simulink model "AdaptiveControlsProjectPart1_Sethi"  (R2019b)
settings: Solver=ode45  StartTime=0.0  StopTime=40  RelTol=1e-6
undefined symbols (not defined in the file): Ar, ar, Astar, astar, B, Br, br, Bstar, bstar, cur0, eps_th, Gam_r, gam_r, Gam_x, gam_x, J, K, L, P, P2, Q, R, th_max, thr0, thx0, Tr_star, tr_star, Tx_star, tx_star, V0, X0, x0, Xr0, xr0
settings Model: Creator=aleon  LastModifiedBy=Japnit Sethi
settings SFSimCC: CustomCodeUndefinedFunction=UseInterfaceOnly

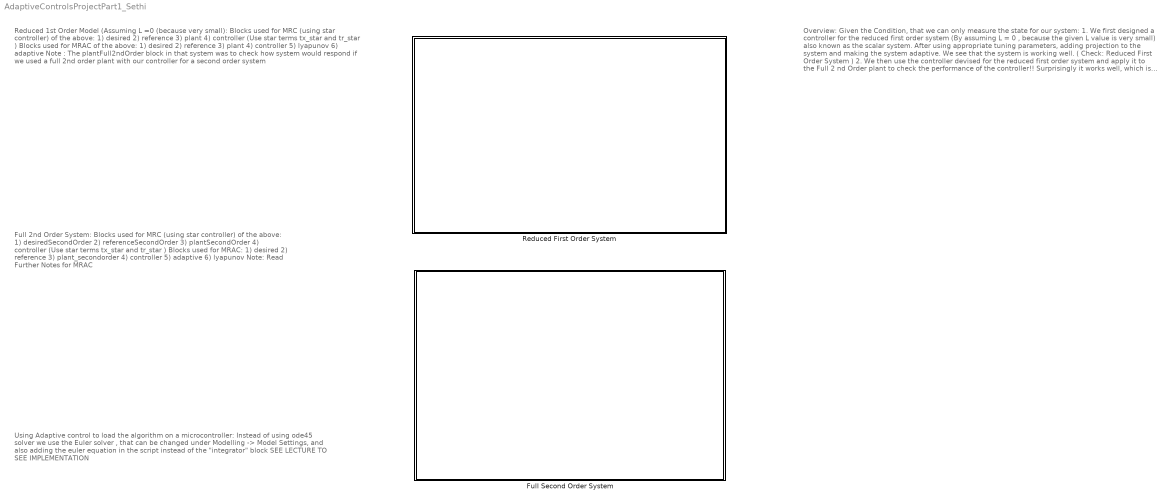
== system AdaptiveControlsProjectPart1_Sethi ==
  note: Reduced 1st Order Model (Assuming L =0 (because very small):
      |
      | Blocks used for MRC (using star controller) of the above:
      | 1) desired
      | 2) reference
      | 3) plant
      | 4) controller (Use star terms tx_star and tr_star )
      |
      | Blocks used for MRAC of the above:
      | 1) desired
      | 2) reference
      | 3) plant
      | 4) controller
      | 5) lyapunov
      | 6) adaptive
      |
      | Note : The plantFull2ndOrder block in that system was to check how system would respond if we used a full 2nd order plant with our controller for a second order system
  note: Using Adaptive control to load the algorithm on a microcontroller:
      |
      | Instead of using ode45 solver we use the Euler solver , that can be changed under Modelling -> Model Settings,
      | and also adding the euler equation in the script instead of the "integrator" block
      |
      | SEE LECTURE TO SEE IMPLEMENTATION
  note: Full 2nd Order System:
      |
      | Blocks used for MRC (using star controller) of the above:
      | 1) desiredSecondOrder
      | 2) referenceSecondOrder
      | 3) plantSecondOrder
      | 4) controller (Use star terms tx_star and tr_star )
      |
      | Blocks used for MRAC:
      | 1) desired
      | 2) reference
      | 3) plant_secondorder
      | 4) controller
      | 5) adaptive
      | 6) lyapunov
      | Note: Read Further Notes for MRAC
  note: Overview:
      | Given the Condition, that we can only measure the state for our system:
      | 1. We first designed a controller for the reduced first order system (By assuming L = 0 , because the given L value is very small) also known as the scalar system. After using appropriate tuning parameters, adding projection to the system and making the system adaptive. We see that the system is working well. ( Check: Reduced First Order System )
      | 2. We then use the controller devised for the reduced first order system and apply it to the Full 2 nd Order plant to check the performance of the controller!! Surprisingly it works well, which is because the approximation of L was legible.
      | 3. We designed a Full state feedback controller for the Full second order system, by deriving the equations in canonical form and also change our states from and to and which is important in order to derive and satisfy our compatibility equations. In this scenario, we were able to measure both and . ( Check: Full Second Order System )
      | 4. Finally, we designed a Full Output Feedback controller , because in really, we cannot measure , the only measurement available to us is .
      | Note: ( Option 2: But not recommended ) For the Full output feedback controller above, we could measure and then calculate the by computing a numerical derivative of measured and adding a filter transfer function to get rid of the noise. But this is not preferred because excessive time that we can lose tuning our parameters to get rid of high oscillations and noise.
  Full Second Order System : Subsystem
  Reduced First Order System : Subsystem

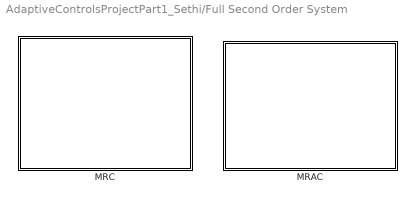
== system AdaptiveControlsProjectPart1_Sethi/Full Second Order System ==
  MRAC : Subsystem
  MRC : Subsystem

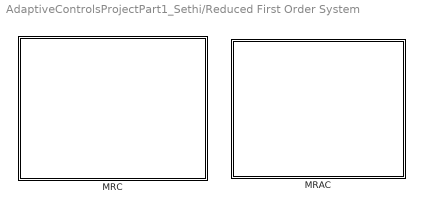
== system AdaptiveControlsProjectPart1_Sethi/Reduced First Order System ==
  MRAC : Subsystem
  MRC : Subsystem

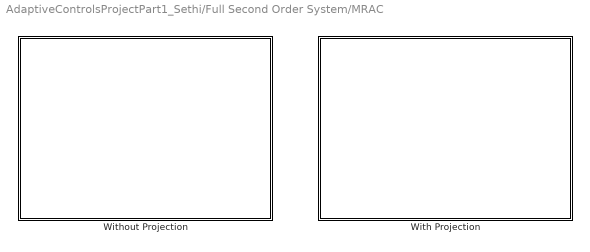
== system AdaptiveControlsProjectPart1_Sethi/Full Second Order System/MRAC ==
  With Projection : Subsystem
  Without Projection : Subsystem

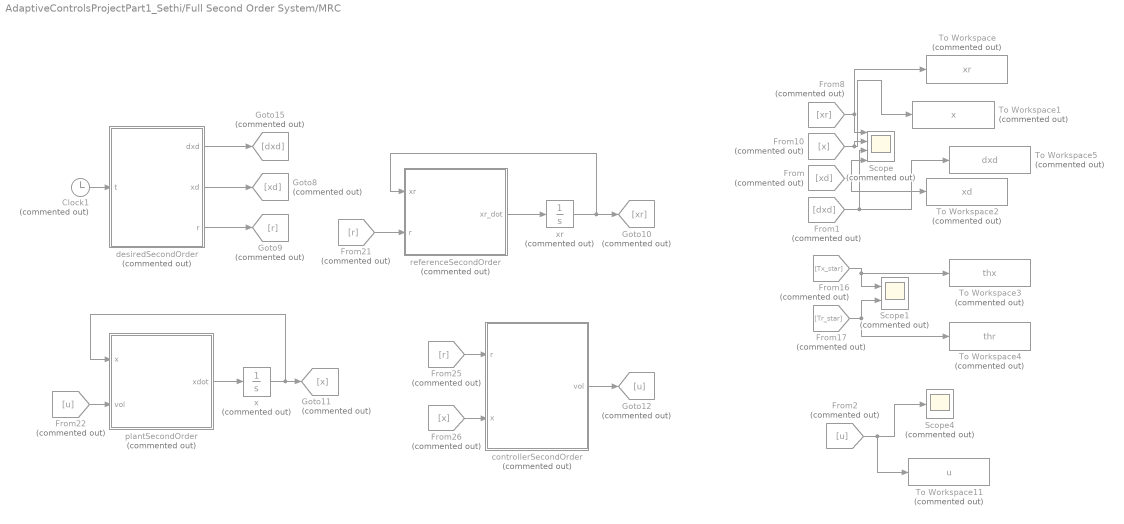
== system AdaptiveControlsProjectPart1_Sethi/Full Second Order System/MRC ==
  Clock1 : Clock  Commented=on
  From : From  Commented=on  GotoTag=xd
  From1 : From  Commented=on  GotoTag=dxd
  From10 : From  Commented=on  GotoTag=x
  From16 : From  Commented=on  GotoTag=Tx_star
  From17 : From  Commented=on  GotoTag=Tr_star
  From2 : From  Commented=on  GotoTag=u
  From21 : From  Commented=on  GotoTag=r
  From22 : From  Commented=on  GotoTag=u
  From25 : From  Commented=on  GotoTag=r
  From26 : From  Commented=on  GotoTag=x
  From8 : From  Commented=on  GotoTag=xr
  Goto10 : Goto  Commented=on  GotoTag=xr
  Goto11 : Goto  Commented=on  GotoTag=x
  Goto12 : Goto  Commented=on  GotoTag=u
  Goto15 : Goto  Commented=on  GotoTag=dxd
  Goto8 : Goto  Commented=on  GotoTag=xd
  Goto9 : Goto  Commented=on  GotoTag=r
  Scope : Scope  Commented=on  NumInputPorts=4
  Scope1 : Scope  Commented=on  NumInputPorts=2
  Scope4 : Scope  Commented=on
  To Workspace : ToWorkspace  Commented=on  VariableName=xr  SampleTime=-1
  To Workspace1 : ToWorkspace  Commented=on  VariableName=x  SampleTime=-1
  To Workspace11 : ToWorkspace  Commented=on  VariableName=u  SampleTime=-1
  To Workspace2 : ToWorkspace  Commented=on  VariableName=xd  SampleTime=-1
  To Workspace3 : ToWorkspace  Commented=on  VariableName=thx  SampleTime=-1
  To Workspace4 : ToWorkspace  Commented=on  VariableName=thr  SampleTime=-1
  To Workspace5 : ToWorkspace  Commented=on  VariableName=dxd  SampleTime=-1
  controllerSecondOrder : MATLAB Function  Commented=on  TreatAsAtomicUnit=on
  desiredSecondOrder : MATLAB Function  Commented=on  TreatAsAtomicUnit=on
  plantSecondOrder : MATLAB Function  Commented=on  TreatAsAtomicUnit=on
  referenceSecondOrder : MATLAB Function  Commented=on  TreatAsAtomicUnit=on
  x : Integrator  Commented=on  InitialCondition=X0
  xr : Integrator  Commented=on  InitialCondition=Xr0
  wires:
  desiredSecondOrder/3(r) -> Goto9/1
  From/1 -> To Workspace2/1, Scope/4
  From1/1 -> To Workspace5/1, Scope/3
  From10/1 -> To Workspace1/1, Scope/2
  x/1 -> plantSecondOrder/1(x), Goto11/1
  controllerSecondOrder/1(vol) -> Goto12/1
  From17/1 -> Scope1/2, To Workspace4/1
  From22/1 -> plantSecondOrder/2(vol)
  desiredSecondOrder/1(dxd) -> Goto15/1
  From26/1 -> controllerSecondOrder/2(x)
  Clock1/1 -> desiredSecondOrder/1(t)
  referenceSecondOrder/1(xr_dot) -> xr/1
  xr/1 -> Goto10/1, referenceSecondOrder/1(xr)
  From8/1 -> Scope/1, To Workspace/1
  From25/1 -> controllerSecondOrder/1(r)
  plantSecondOrder/1(xdot) -> x/1
  desiredSecondOrder/2(xd) -> Goto8/1
  From21/1 -> referenceSecondOrder/2(r)
  From16/1 -> To Workspace3/1, Scope1/1
  From2/1 -> To Workspace11/1, Scope4/1

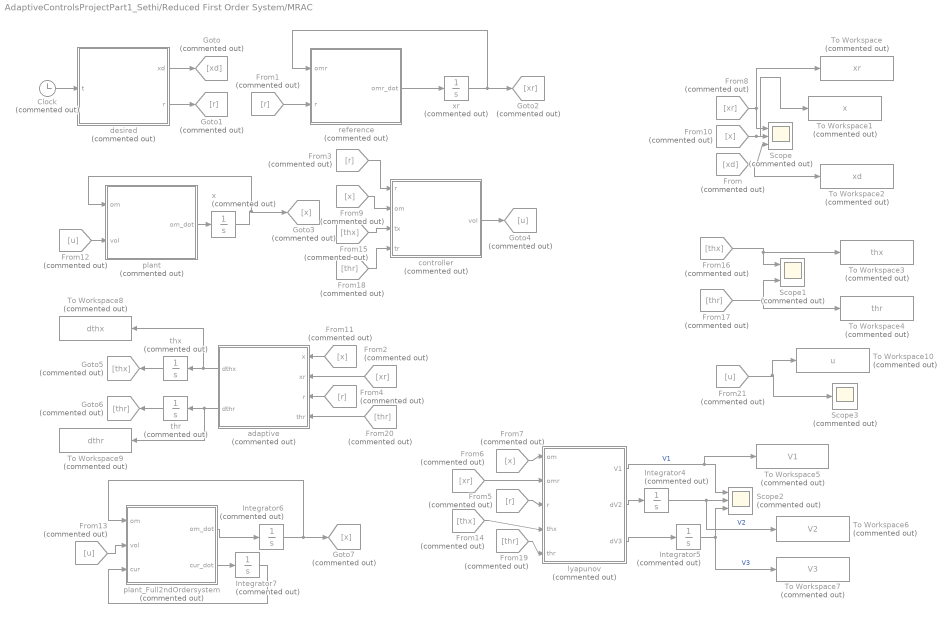
== system AdaptiveControlsProjectPart1_Sethi/Reduced First Order System/MRAC ==
  Clock : Clock  Commented=on
  From : From  Commented=on  GotoTag=xd
  From{1,3..5} (4 alike) : From  Commented=on  GotoTag=r
  From{7,9..11} (4 alike) : From  Commented=on  GotoTag=x
  From12 : From  Commented=on  GotoTag=u
  From13 : From  Commented=on  GotoTag=u
  From14 : From  Commented=on  GotoTag=thx
  From15 : From  Commented=on  GotoTag=thx
  From16 : From  Commented=on  GotoTag=thx
  From{17..20} (4 alike) : From  Commented=on  GotoTag=thr
  From2 : From  Commented=on  GotoTag=xr
  From21 : From  Commented=on  GotoTag=u
  From6 : From  Commented=on  GotoTag=xr
  From8 : From  Commented=on  GotoTag=xr
  Goto : Goto  Commented=on  GotoTag=xd
  Goto1 : Goto  Commented=on  GotoTag=r
  Goto2 : Goto  Commented=on  GotoTag=xr
  Goto3 : Goto  Commented=on  GotoTag=x
  Goto4 : Goto  Commented=on  GotoTag=u
  Goto5 : Goto  Commented=on  GotoTag=thx
  Goto6 : Goto  Commented=on  GotoTag=thr
  Goto7 : Goto  Commented=on  GotoTag=x
  Integrator4 : Integrator  Commented=on  InitialCondition=V0
  Integrator5 : Integrator  Commented=on  InitialCondition=V0
  Integrator6 : Integrator  Commented=on  InitialCondition=x0
  Integrator7 : Integrator  Commented=on  InitialCondition=cur0
  Scope : Scope  Commented=on  NumInputPorts=3
  Scope1 : Scope  Commented=on  NumInputPorts=2
  Scope2 : Scope  Commented=on  NumInputPorts=3
  Scope3 : Scope  Commented=on
  To Workspace : ToWorkspace  Commented=on  VariableName=xr  SampleTime=-1
  To Workspace1 : ToWorkspace  Commented=on  VariableName=x  SampleTime=-1
  To Workspace10 : ToWorkspace  Commented=on  VariableName=u  SampleTime=-1
  To Workspace2 : ToWorkspace  Commented=on  VariableName=xd  SampleTime=-1
  To Workspace3 : ToWorkspace  Commented=on  VariableName=thx  SampleTime=-1
  To Workspace4 : ToWorkspace  Commented=on  VariableName=thr  SampleTime=-1
  To Workspace5 : ToWorkspace  Commented=on  VariableName=V1  SampleTime=-1
  To Workspace6 : ToWorkspace  Commented=on  VariableName=V2  SampleTime=-1
  To Workspace7 : ToWorkspace  Commented=on  VariableName=V3  SampleTime=-1
  To Workspace8 : ToWorkspace  Commented=on  VariableName=dthx  SampleTime=-1
  To Workspace9 : ToWorkspace  Commented=on  VariableName=dthr  SampleTime=-1
  adaptive : MATLAB Function  Commented=on  TreatAsAtomicUnit=on
  controller : MATLAB Function  Commented=on  TreatAsAtomicUnit=on
  desired : MATLAB Function  Commented=on  TreatAsAtomicUnit=on
  lyapunov : MATLAB Function  Commented=on  TreatAsAtomicUnit=on
  plant : MATLAB Function  Commented=on  TreatAsAtomicUnit=on
  plant_Full2ndOrdersystem : MATLAB Function  Commented=on  TreatAsAtomicUnit=on
  reference : MATLAB Function  Commented=on  TreatAsAtomicUnit=on
  thr : Integrator  Commented=on  InitialCondition=thr0
  thx : Integrator  Commented=on  InitialCondition=thx0
  x : Integrator  Commented=on  InitialCondition=x0
  xr : Integrator  Commented=on  InitialCondition=xr0
  wires:
  From13/1 -> plant_Full2ndOrdersystem/2(vol)
  plant/1(om_dot) -> x/1
  lyapunov/3(dV3) -> Integrator5/1
  From7/1 -> lyapunov/1(om)
  plant_Full2ndOrdersystem/1(om_dot) -> Integrator6/1
  Integrator4/1 -> To Workspace6/1, Scope2/2  "V2"
  xr/1 -> Goto2/1, reference/1(omr)
  From10/1 -> To Workspace1/1, Scope/2
  From11/1 -> adaptive/1(x)
  From6/1 -> lyapunov/2(omr)
  From19/1 -> lyapunov/5(thr)
  From1/1 -> reference/2(r)
  Integrator6/1 -> Goto7/1, plant_Full2ndOrdersystem/1(om)
  reference/1(omr_dot) -> xr/1
  plant_Full2ndOrdersystem/2(cur_dot) -> Integrator7/1
  controller/1(vol) -> Goto4/1
  desired/1(xd) -> Goto/1
  From12/1 -> plant/2(vol)
  Integrator5/1 -> To Workspace7/1, Scope2/3  "V3"
  Clock/1 -> desired/1(t)
  adaptive/1(dthx) -> To Workspace8/1, thx/1
  adaptive/2(dthr) -> To Workspace9/1, thr/1
  From18/1 -> controller/4(tr)
  From16/1 -> To Workspace3/1, Scope1/1
  From4/1 -> adaptive/3(r)
  lyapunov/2(dV2) -> Integrator4/1
  From5/1 -> lyapunov/3(r)
  From2/1 -> adaptive/2(xr)
  lyapunov/1(V1) -> To Workspace5/1, Scope2/1  "V1"
  From8/1 -> Scope/1, To Workspace/1
  From/1 -> To Workspace2/1, Scope/3
  From14/1 -> lyapunov/4(thx)
  From17/1 -> Scope1/2, To Workspace4/1
  From20/1 -> adaptive/4(thr)
  x/1 -> Goto3/1, plant/1(om)
  thr/1 -> Goto6/1
  desired/2(r) -> Goto1/1
  thx/1 -> Goto5/1
  From3/1 -> controller/1(r)
  Integrator7/1 -> plant_Full2ndOrdersystem/3(cur)
  From9/1 -> controller/2(om)
  From15/1 -> controller/3(tx)
  From21/1 -> Scope3/1, To Workspace10/1

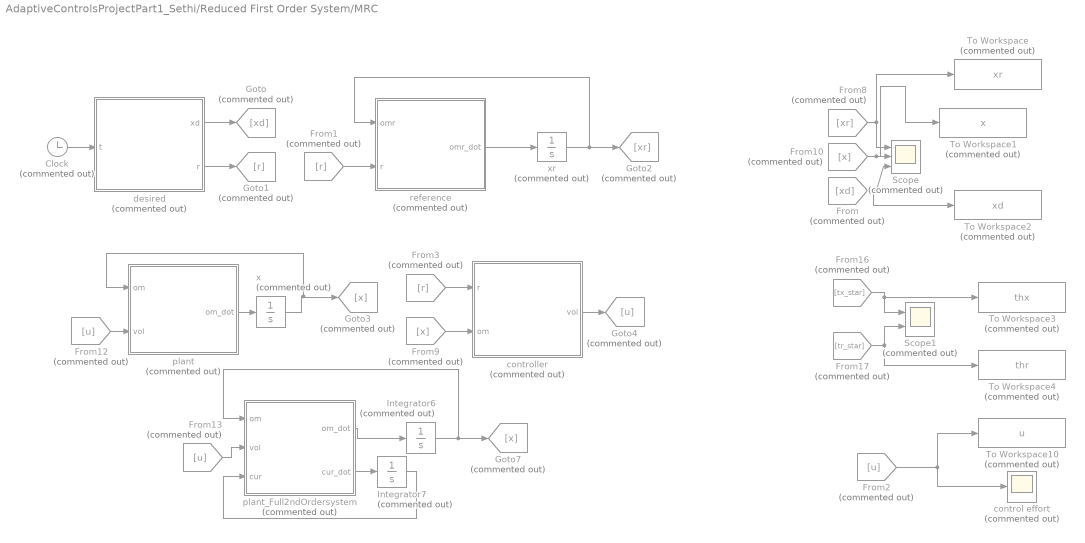
== system AdaptiveControlsProjectPart1_Sethi/Reduced First Order System/MRC ==
  Clock : Clock  Commented=on
  From : From  Commented=on  GotoTag=xd
  From1 : From  Commented=on  GotoTag=r
  From10 : From  Commented=on  GotoTag=x
  From12 : From  Commented=on  GotoTag=u
  From13 : From  Commented=on  GotoTag=u
  From16 : From  Commented=on  GotoTag=tx_star
  From17 : From  Commented=on  GotoTag=tr_star
  From2 : From  Commented=on  GotoTag=u
  From3 : From  Commented=on  GotoTag=r
  From8 : From  Commented=on  GotoTag=xr
  From9 : From  Commented=on  GotoTag=x
  Goto : Goto  Commented=on  GotoTag=xd
  Goto1 : Goto  Commented=on  GotoTag=r
  Goto2 : Goto  Commented=on  GotoTag=xr
  Goto3 : Goto  Commented=on  GotoTag=x
  Goto4 : Goto  Commented=on  GotoTag=u
  Goto7 : Goto  Commented=on  GotoTag=x
  Integrator6 : Integrator  Commented=on  InitialCondition=x0
  Integrator7 : Integrator  Commented=on  InitialCondition=cur0
  Scope : Scope  Commented=on  NumInputPorts=3
  Scope1 : Scope  Commented=on  NumInputPorts=2
  To Workspace : ToWorkspace  Commented=on  VariableName=xr  SampleTime=-1
  To Workspace1 : ToWorkspace  Commented=on  VariableName=x  SampleTime=-1
  To Workspace10 : ToWorkspace  Commented=on  VariableName=u  SampleTime=-1
  To Workspace2 : ToWorkspace  Commented=on  VariableName=xd  SampleTime=-1
  To Workspace3 : ToWorkspace  Commented=on  VariableName=thx  SampleTime=-1
  To Workspace4 : ToWorkspace  Commented=on  VariableName=thr  SampleTime=-1
  control effort : Scope  Commented=on
  controller : MATLAB Function  Commented=on  TreatAsAtomicUnit=on
  desired : MATLAB Function  Commented=on  TreatAsAtomicUnit=on
  plant : MATLAB Function  Commented=on  TreatAsAtomicUnit=on
  plant_Full2ndOrdersystem : MATLAB Function  Commented=on  TreatAsAtomicUnit=on
  reference : MATLAB Function  Commented=on  TreatAsAtomicUnit=on
  x : Integrator  Commented=on  InitialCondition=x0
  xr : Integrator  Commented=on  InitialCondition=xr0
  wires:
  controller/1(vol) -> Goto4/1
  desired/2(r) -> Goto1/1
  From9/1 -> controller/2(om)
  Clock/1 -> desired/1(t)
  From12/1 -> plant/2(vol)
  x/1 -> Goto3/1, plant/1(om)
  From3/1 -> controller/1(r)
  desired/1(xd) -> Goto/1
  reference/1(omr_dot) -> xr/1
  xr/1 -> Goto2/1, reference/1(omr)
  plant/1(om_dot) -> x/1
  From1/1 -> reference/2(r)
  From17/1 -> Scope1/2, To Workspace4/1
  From/1 -> To Workspace2/1, Scope/3
  From8/1 -> Scope/1, To Workspace/1
  From16/1 -> To Workspace3/1, Scope1/1
  From10/1 -> To Workspace1/1, Scope/2
  Integrator6/1 -> Goto7/1, plant_Full2ndOrdersystem/1(om)
  plant_Full2ndOrdersystem/2(cur_dot) -> Integrator7/1
  Integrator7/1 -> plant_Full2ndOrdersystem/3(cur)
  From13/1 -> plant_Full2ndOrdersystem/2(vol)
  plant_Full2ndOrdersystem/1(om_dot) -> Integrator6/1
  From2/1 -> control effort/1, To Workspace10/1

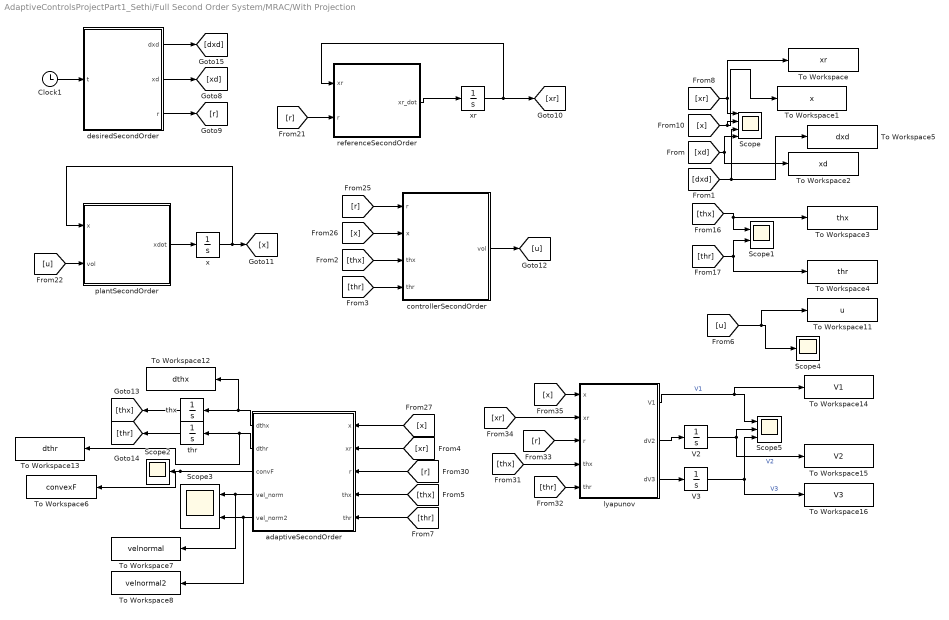
== system AdaptiveControlsProjectPart1_Sethi/Full Second Order System/MRAC/With Projection ==
  Clock1 : Clock
  Scope : Scope  NumInputPorts=4
  Scope1 : Scope  NumInputPorts=2
  Scope2 : Scope
  Scope3 : Scope  NumInputPorts=2
  Scope4 : Scope
  Scope5 : Scope  NumInputPorts=3
  To Workspace : ToWorkspace  VariableName=xr  SampleTime=-1
  To Workspace1 : ToWorkspace  VariableName=x  SampleTime=-1
  To Workspace11 : ToWorkspace  VariableName=u  SampleTime=-1
  To Workspace12 : ToWorkspace  VariableName=dthx  SampleTime=-1
  To Workspace13 : ToWorkspace  VariableName=dthr  SampleTime=-1
  To Workspace14 : ToWorkspace  VariableName=V1  SampleTime=-1
  To Workspace15 : ToWorkspace  VariableName=V2  SampleTime=-1
  To Workspace16 : ToWorkspace  VariableName=V3  SampleTime=-1
  To Workspace2 : ToWorkspace  VariableName=xd  SampleTime=-1
  To Workspace3 : ToWorkspace  VariableName=thx  SampleTime=-1
  To Workspace4 : ToWorkspace  VariableName=thr  SampleTime=-1
  To Workspace5 : ToWorkspace  VariableName=dxd  SampleTime=-1
  To Workspace6 : ToWorkspace  VariableName=convexF  SaveFormat=Timeseries  SampleTime=-1
  To Workspace7 : ToWorkspace  VariableName=velnormal  SaveFormat=Timeseries  SampleTime=-1
  To Workspace8 : ToWorkspace  VariableName=velnormal2  SaveFormat=Timeseries  SampleTime=-1
  V2 : Integrator  InitialCondition=V0
  V3 : Integrator  InitialCondition=V0
  adaptiveSecondOrder : MATLAB Function  TreatAsAtomicUnit=on
  controllerSecondOrder : MATLAB Function  TreatAsAtomicUnit=on
  desiredSecondOrder : MATLAB Function  TreatAsAtomicUnit=on
  lyapunov : MATLAB Function  TreatAsAtomicUnit=on
  plantSecondOrder : MATLAB Function  TreatAsAtomicUnit=on
  referenceSecondOrder : MATLAB Function  TreatAsAtomicUnit=on
  thr : Integrator  InitialCondition=thr0
  thx : Integrator  InitialCondition=thx0
  x : Integrator  InitialCondition=X0
  xr : Integrator  InitialCondition=Xr0
  wires:
  [dxd] -> To Workspace5/1, Scope/3
  [thx] -> To Workspace3/1, Scope1/1
  xr/1 -> [xr], referenceSecondOrder/1(xr)
  V2/1 -> Scope5/2, To Workspace15/1  "V2"
  lyapunov/3(dV3) -> V3/1
  [thr] -> adaptiveSecondOrder/5(thr)
  [x] -> lyapunov/1(x)
  lyapunov/2(dV2) -> V2/1
  [r] -> controllerSecondOrder/1(r)
  [xd] -> To Workspace2/1, Scope/4
  [xr] -> Scope/1, To Workspace/1
  [thx] -> adaptiveSecondOrder/4(thx)
  adaptiveSecondOrder/4(vel_norm) -> To Workspace7/1, Scope3/1
  thr/1 -> [thr]
  adaptiveSecondOrder/5(vel_norm2) -> To Workspace8/1, Scope3/2
  [r] -> adaptiveSecondOrder/3(r)
  adaptiveSecondOrder/3(convF) -> To Workspace6/1, Scope2/1
  Clock1/1 -> desiredSecondOrder/1(t)
  desiredSecondOrder/3(r) -> [r]
  [xr] -> lyapunov/2(xr)
  x/1 -> plantSecondOrder/1(x), [x]
  [x] -> To Workspace1/1, Scope/2
  [thr] -> lyapunov/5(thr)
  [x] -> controllerSecondOrder/2(x)
  adaptiveSecondOrder/2(dthr) -> To Workspace13/1, thr/1
  [thr] -> Scope1/2, To Workspace4/1
  [thx] -> controllerSecondOrder/3(thx)
  referenceSecondOrder/1(xr_dot) -> xr/1
  V3/1 -> Scope5/3, To Workspace16/1  "V3"
  plantSecondOrder/1(xdot) -> x/1
  desiredSecondOrder/2(xd) -> [xd]
  [u] -> To Workspace11/1, Scope4/1
  [thr] -> controllerSecondOrder/4(thr)
  [thx] -> lyapunov/4(thx)
  desiredSecondOrder/1(dxd) -> [dxd]
  [x] -> adaptiveSecondOrder/1(x)
  controllerSecondOrder/1(vol) -> [u]
  thx/1 -> [thx]
  lyapunov/1(V1) -> To Workspace14/1, Scope5/1  "V1"
  [u] -> plantSecondOrder/2(vol)
  [r] -> lyapunov/3(r)
  [xr] -> adaptiveSecondOrder/2(xr)
  [r] -> referenceSecondOrder/2(r)
  adaptiveSecondOrder/1(dthx) -> To Workspace12/1, thx/1

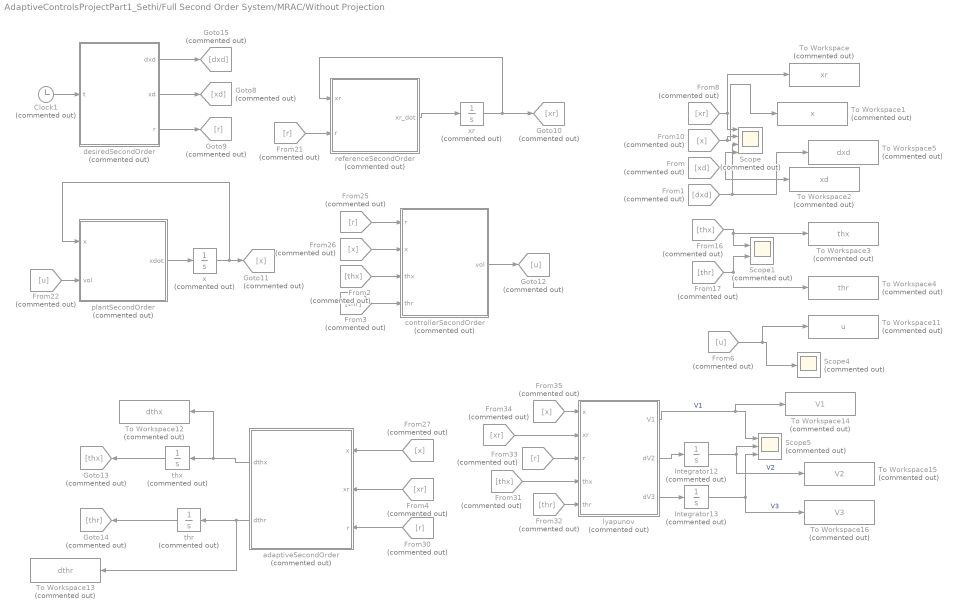
== system AdaptiveControlsProjectPart1_Sethi/Full Second Order System/MRAC/Without Projection ==
  Clock1 : Clock  Commented=on
  From : From  Commented=on  GotoTag=xd
  From1 : From  Commented=on  GotoTag=dxd
  From{10,26..27,35} (4 alike) : From  Commented=on  GotoTag=x
  From16 : From  Commented=on  GotoTag=thx
  From17 : From  Commented=on  GotoTag=thr
  From2 : From  Commented=on  GotoTag=thx
  From{21,25,30,33} (4 alike) : From  Commented=on  GotoTag=r
  From22 : From  Commented=on  GotoTag=u
  From3 : From  Commented=on  GotoTag=thr
  From31 : From  Commented=on  GotoTag=thx
  From32 : From  Commented=on  GotoTag=thr
  From34 : From  Commented=on  GotoTag=xr
  From4 : From  Commented=on  GotoTag=xr
  From6 : From  Commented=on  GotoTag=u
  From8 : From  Commented=on  GotoTag=xr
  Goto10 : Goto  Commented=on  GotoTag=xr
  Goto11 : Goto  Commented=on  GotoTag=x
  Goto12 : Goto  Commented=on  GotoTag=u
  Goto13 : Goto  Commented=on  GotoTag=thx
  Goto14 : Goto  Commented=on  GotoTag=thr
  Goto15 : Goto  Commented=on  GotoTag=dxd
  Goto8 : Goto  Commented=on  GotoTag=xd
  Goto9 : Goto  Commented=on  GotoTag=r
  Integrator12 : Integrator  Commented=on  InitialCondition=V0
  Integrator13 : Integrator  Commented=on  InitialCondition=V0
  Scope : Scope  Commented=on  NumInputPorts=4
  Scope1 : Scope  Commented=on  NumInputPorts=2
  Scope4 : Scope  Commented=on
  Scope5 : Scope  Commented=on  NumInputPorts=3
  To Workspace : ToWorkspace  Commented=on  VariableName=xr  SampleTime=-1
  To Workspace1 : ToWorkspace  Commented=on  VariableName=x  SampleTime=-1
  To Workspace11 : ToWorkspace  Commented=on  VariableName=u  SampleTime=-1
  To Workspace12 : ToWorkspace  Commented=on  VariableName=dthx  SampleTime=-1
  To Workspace13 : ToWorkspace  Commented=on  VariableName=dthr  SampleTime=-1
  To Workspace14 : ToWorkspace  Commented=on  VariableName=V1  SampleTime=-1
  To Workspace15 : ToWorkspace  Commented=on  VariableName=V2  SampleTime=-1
  To Workspace16 : ToWorkspace  Commented=on  VariableName=V3  SampleTime=-1
  To Workspace2 : ToWorkspace  Commented=on  VariableName=xd  SampleTime=-1
  To Workspace3 : ToWorkspace  Commented=on  VariableName=thx  SampleTime=-1
  To Workspace4 : ToWorkspace  Commented=on  VariableName=thr  SampleTime=-1
  To Workspace5 : ToWorkspace  Commented=on  VariableName=dxd  SampleTime=-1
  adaptiveSecondOrder : MATLAB Function  Commented=on  TreatAsAtomicUnit=on
  controllerSecondOrder : MATLAB Function  Commented=on  TreatAsAtomicUnit=on
  desiredSecondOrder : MATLAB Function  Commented=on  TreatAsAtomicUnit=on
  lyapunov : MATLAB Function  Commented=on  TreatAsAtomicUnit=on
  plantSecondOrder : MATLAB Function  Commented=on  TreatAsAtomicUnit=on
  referenceSecondOrder : MATLAB Function  Commented=on  TreatAsAtomicUnit=on
  thr : Integrator  Commented=on  InitialCondition=thr0
  thx : Integrator  Commented=on  InitialCondition=thx0
  x : Integrator  Commented=on  InitialCondition=X0
  xr : Integrator  Commented=on  InitialCondition=Xr0
  wires:
  From1/1 -> To Workspace5/1, Scope/3
  From16/1 -> To Workspace3/1, Scope1/1
  xr/1 -> Goto10/1, referenceSecondOrder/1(xr)
  Integrator12/1 -> Scope5/2, To Workspace15/1  "V2"
  lyapunov/3(dV3) -> Integrator13/1
  From35/1 -> lyapunov/1(x)
  lyapunov/2(dV2) -> Integrator12/1
  From25/1 -> controllerSecondOrder/1(r)
  From/1 -> To Workspace2/1, Scope/4
  From8/1 -> Scope/1, To Workspace/1
  thr/1 -> Goto14/1
  From30/1 -> adaptiveSecondOrder/3(r)
  Clock1/1 -> desiredSecondOrder/1(t)
  desiredSecondOrder/3(r) -> Goto9/1
  From34/1 -> lyapunov/2(xr)
  x/1 -> plantSecondOrder/1(x), Goto11/1
  From10/1 -> To Workspace1/1, Scope/2
  From32/1 -> lyapunov/5(thr)
  From26/1 -> controllerSecondOrder/2(x)
  adaptiveSecondOrder/2(dthr) -> thr/1, To Workspace13/1
  From17/1 -> Scope1/2, To Workspace4/1
  From2/1 -> controllerSecondOrder/3(thx)
  referenceSecondOrder/1(xr_dot) -> xr/1
  Integrator13/1 -> Scope5/3, To Workspace16/1  "V3"
  plantSecondOrder/1(xdot) -> x/1
  desiredSecondOrder/2(xd) -> Goto8/1
  From6/1 -> To Workspace11/1, Scope4/1
  From3/1 -> controllerSecondOrder/4(thr)
  From31/1 -> lyapunov/4(thx)
  desiredSecondOrder/1(dxd) -> Goto15/1
  From27/1 -> adaptiveSecondOrder/1(x)
  controllerSecondOrder/1(vol) -> Goto12/1
  thx/1 -> Goto13/1
  lyapunov/1(V1) -> To Workspace14/1, Scope5/1  "V1"
  From22/1 -> plantSecondOrder/2(vol)
  From33/1 -> lyapunov/3(r)
  From4/1 -> adaptiveSecondOrder/2(xr)
  From21/1 -> referenceSecondOrder/2(r)
  adaptiveSecondOrder/1(dthx) -> To Workspace12/1, thx/1

== matlab function AdaptiveControlsProjectPart1_Sethi/Reduced First Order System/MRAC/reference ==
  data: omr input; omr_dot output; r input; ar parameter; br parameter
function omr_dot = reference(omr,r,ar, br)

omr_dot = ar*omr + br*r;

== matlab function AdaptiveControlsProjectPart1_Sethi/Reduced First Order System/MRAC/plant ==
  data: om input; om_dot output; vol input; astar parameter; bstar parameter
function om_dot = plant(om,vol,astar, bstar)

om_dot = astar*om + bstar*vol;

== matlab function AdaptiveControlsProjectPart1_Sethi/Reduced First Order System/MRAC/desired ==
  data: xd output; t input; r output; ar parameter; br parameter
function [xd,r] = desired(t,ar, br)

xd = 10*sin(2*t);
dxd = 20*cos(2*t);

r = (dxd - ar*xd)/br;

== matlab function AdaptiveControlsProjectPart1_Sethi/Reduced First Order System/MRAC/controller ==
  data: r input; om input; vol output; tx input; tr input
%%%%%%%%%%%%%%%%%%%%%%%%%%%%%%%%%%%%%%%%%%%%%%%%%%%%%%%%%%%%%%%%%%%%%%%%%
%--- MRC, using star Controller (Without making the system adaptive) ---%
%%%%%%%%%%%%%%%%%%%%%%%%%%%%%%%%%%%%%%%%%%%%%%%%%%%%%%%%%%%%%%%%%%%%%%%%%
function vol = controller(r,om,tx, tr)
vol = tx*om + tr*r;

== matlab function AdaptiveControlsProjectPart1_Sethi/Reduced First Order System/MRAC/adaptive ==
  data: x input; xr input; r input; thr input; dthx output; dthr output; gam_x parameter; gam_r parameter; bstar parameter
function [dthx,dthr] = adaptive(x,xr,r,thr,gam_x, gam_r, bstar)
% Adaptive Control Update Law
% Error dynamics
e = x - xr;

% Theta_x_dot and Theta_r_dot
dthx = -sign(bstar)*gam_x*x*e;
dthr = -sign(bstar)*gam_r*r*e;

% To set a saturation limit, theta_r star is 0.1161
if thr<0.01 && dthr<0, dthr=0; end

== matlab function AdaptiveControlsProjectPart1_Sethi/Reduced First Order System/MRAC/lyapunov ==
  data: om input; omr input; r input; V1 output; thx input; thr input; dV2 output; dV3 output; gam_x parameter; gam_r parameter; tx_star parameter; tr_star parameter; ar parameter; br parameter; astar parameter; bstar parameter
function [V1,dV2,dV3] = lyapunov(om,omr,r,thx,thr,gam_x, gam_r, tx_star, tr_star,ar, br, astar, bstar)

e = om - omr;
dV3= ar*e^2;


dthx = -sign(bstar)*gam_x*om*e;
dthr = -sign(bstar)*gam_r*r*e;

% Projection (Mainly to set a saturation limit)
% theta_r < 0.01 (threshold) and dtheta_r < 0 (making theta_r even more
% negative), which we want to avoid
if thr<0.01 && dthr<0
    dthr=0; 
    dV3= ar*e^2 + abs(bstar)*(thr - tr_star)*(sign(bstar)*r*e + dthr/gam_r);
end

vol = thx*om + thr*r;

omr_dot = ar*omr + br*r; 
om_dot = astar*om + bstar*vol; 
edot= om_dot - omr_dot;

V1 = .5*e^2 + .5*abs(bstar)/gam_x*(thx - tx_star)^2 + .5*abs(bstar)/gam_r*(thr - tr_star)^2;
dV2= e*edot + abs(bstar)/gam_x*(thx - tx_star)*dthx + abs(bstar)/gam_r*(thr - tr_star)*dthr;

== matlab function AdaptiveControlsProjectPart1_Sethi/Reduced First Order System/MRAC/plant_Full2ndOrdersystem ==
  data: om input; om_dot output; vol input; J parameter; cur_dot output; B parameter; K parameter; L parameter; R parameter; cur input
function [om_dot, cur_dot] = plant(om,vol, J, B, K, L, R, cur)
% This is Assuming we did not know that Plant could be reduced to 1st order
% So we apply the full2nd order dynamic system in place of an approximated
% system
% Second order system !! Not assuming L = 0
om_dot = 1/J*(-B*om + K*cur);
cur_dot = 1/L*(-K*om - R*cur + vol);

% Note: The gains that worked for me were:
% ar = -10;   
% br = 10;
% 
% gam_x = 0.1;
% gam_r = 0.1;
% But obviously the theta_x and theta_r do not converge because I built a
% controller for a 1st order system but closing the loop with 2nd order
% system
% And you would notice that in the actual and reference trajectory graph
% that it never converges at some points, which most probably are the
% points where we have neglected L since it is too small but maybe the
% di/dt value is too large that it punishes us for our assumption of
% neglecting L

== matlab function AdaptiveControlsProjectPart1_Sethi/Full Second Order System/MRC/desiredSecondOrder ==
  data: dxd output; xd output; t input; r output; Ar parameter; Br parameter
function [dxd, xd,r] = desiredSecondOrder(t,Ar, Br)
xd = 10*sin(2*t);
dxd = 20*cos(2*t);
ddxd = -40*sin(2*t);

% r = (ddxd - ar1*xd - ar2*dxd)/br;
r = (ddxd - Ar(2,1)*xd - Ar(2,2)*dxd)/Br(2,1);

== matlab function AdaptiveControlsProjectPart1_Sethi/Full Second Order System/MRC/referenceSecondOrder ==
  data: xr input; xr_dot output; r input; Ar parameter; Br parameter
function xr_dot = referenceSecondOrder(xr, r, Ar, Br)

% xr_dot = [0, 1; ar1, ar2]*xr + [0; br]*r;
xr_dot = Ar*xr + Br*r;

== matlab function AdaptiveControlsProjectPart1_Sethi/Full Second Order System/MRC/plantSecondOrder ==
  data: x input; xdot output; vol input; Astar parameter; Bstar parameter
%%%%%%%%%%%%%%%%%%%%%%%%%%%%%%%%%%%%%%%%%%%%%%%%%%%%%%%%%%%%%%%%%%%%%%%%%
%--- MRC, using star Controller (Without making the system adaptive) ---%
%%%%%%%%%%%%%%%%%%%%%%%%%%%%%%%%%%%%%%%%%%%%%%%%%%%%%%%%%%%%%%%%%%%%%%%%%

function xdot  = plantSecondOrder(x,vol, Astar, Bstar)
% Note: vol is your control effort u
xdot = Astar*x + Bstar*vol;  % xdot = [0, 1; astar1 astar2]*x + [0; bstar]*vol;
%om_dot = [1 0]*xdot;

== matlab function AdaptiveControlsProjectPart1_Sethi/Full Second Order System/MRC/controllerSecondOrder ==
  data: r input; x input; vol output; Tx_star parameter; Tr_star parameter
%%%%%%%%%%%%%%%%%%%%%%%%%%%%%%%%%%%%%%%%%%%%%%%%%%%%%%%%%%%%%%%%%%%%%%%%%
%--- MRC, using star Controller (Without making the system adaptive) ---%
%%%%%%%%%%%%%%%%%%%%%%%%%%%%%%%%%%%%%%%%%%%%%%%%%%%%%%%%%%%%%%%%%%%%%%%%%
function vol = controller(r,x,Tx_star, Tr_star)
% % vol = [Tx_star1 Tx_star2]'*X + Tr_star*r;     
vol = Tx_star'*x + Tr_star*r;   % Do not forget the transpose sign for Tx_star'
% % Note: Tx_star and Tr_star are your constant parameters from the main .m
% % script taken in the simulink model !!! So do not forget to change both
% % Tx_star and Tr_star to be taken as parameters in the "Model Explorer" in
% % Simulink

% % Note: The gains that worked for me were:
% ar1 = -50; % Just tune these values
% ar2 = -40; % Just tune these values
% br = 10;
% Ar = [0, 1; ar1, ar2];   
% Br = [0; br];

== matlab function AdaptiveControlsProjectPart1_Sethi/Full Second Order System/MRAC/With Projection/adaptiveSecondOrder ==
  data: x input; xr input; r input; Gam_x parameter; Gam_r parameter; Bstar parameter; dthx output; dthr output; P2 parameter; thx input; thr input; convF output; vel_norm output; vel_norm2 output; eps_th parameter; th_max parameter

%%%%%%%%%%%%%%%%%%%%%%%%%%%%
%------WITH PROJECTION-----%
%%%%%%%%%%%%%%%%%%%%%%%%%%%%

function [dthx,dthr, convF,vel_norm, vel_norm2] =...
    adaptiveSecondOrder(x, xr, r,Gam_x, Gam_r, Bstar, P2, thx, thr, eps_th, th_max)
% Adaptive Control Update Law
% Error dynamics
e = x - xr;

% % Theta_x_dot and Theta_r_dot
% % Note: Need to put e'*P2 in parenthesis because the result is a scalar and
% % I want Matlab to multiple that scalar to Gam_x matrix and not Gam_x
% % matrix to the vector e' first !!!
dthx = -Gam_x*(e'*P2)*x*sign(Bstar(2,1)); % dThx = -Gam_x*e'*P2*x*sign(bstar);
dthr = -Gam_r*(e'*P2)*r*sign(Bstar(2,1)); % dThr = -Gam_r*e'*P2*r*sign(bstar);

%%%%%%%%%%%%%%%%%%%%%%%%%%%%%%%%%%%%%%%%%%%
%------ Projection Algorithm Stuff  -----%
%%%%%%%%%%%%%%%%%%%%%%%%%%%%%%%%%%%%%%%%%%%
theta = [thx; thr];
dtheta = [dthx; dthr];

% Smooth Convex Function Pg. 121 "Adaptive Control Notes"
convF = (theta'*theta - th_max^2)/(eps_th*th_max^2); % Circular Convex Set
% We can make different shapes of convex sets. For example if we add a
% matrix M in between like convF = (theta'*M*theta -
% th_max^2)/(eps_th*th_max^2); we can make it a eliptical convex set

gradf = 2*theta/(eps_th*th_max^2);
gradf_norm = gradf/norm(gradf); % Normalized Gradient = Grad_f/norm of Grad_f

% Note: vel is theta_dot
vel_norm = dtheta'*gradf_norm;  % Normal Velocity vector, This is before saturation
vel_norm2 = vel_norm; % 

% If I am outside the region
if convF>0 && vel_norm>0    % if Velocity normal is pointing outside then you take away a little bit of velocity
   new_dtheta = dtheta - gradf_norm*vel_norm*convF; % 3rd part of Eq. (203) Pg. 121 "Adaptive Control Notes"
   dthx = new_dtheta(1:2);
   dthr = new_dtheta(3);
   vel_norm2 = new_dtheta'*gradf_norm; % Computed New velocity normal to compare with vel_norm !! Just to see how effective the algorithm was
   % Don't really need vel_norm2, just for comparison purpose
   % vel_norm2 is after SATURATION % after Projection is applied
end

== matlab function AdaptiveControlsProjectPart1_Sethi/Full Second Order System/MRAC/With Projection/lyapunov ==
  data: x input; xr input; r input; V1 output; thx input; thr input; dV2 output; dV3 output; P parameter; Q parameter; Gam_x parameter; Gam_r parameter; Astar parameter; Br parameter; Tx_star parameter; Tr_star parameter; Bstar parameter; Ar parameter
function [V1,dV2,dV3] = lyapunov(x,xr,r,thx,thr,P,Q,Gam_x,Gam_r,...
                                 Astar,Br,Tx_star, Tr_star, Bstar, Ar)

P2 = P(:,2);

e = x - xr;
dV3= -e'*Q*e;

dthx = -Gam_x*(e'*P2)*x*sign(Bstar(2,1)); % -Gam_x*(e'*P2)*x*sign(bstar);
dthr = -Gam_r*(e'*P2)*r*sign(Bstar(2,1)); % -gam_r*(e'*P2)*r*sign(bstar);

vol = thx'*x + thr*r;
 
xr_dot = Ar*xr + Br*r;    % Ar*xr + [0 ; br]*r; 
x_dot = Astar*x + Bstar*vol; % [0 1;astar1 astar2]*x + [0 ; bstar]*vol;
edot= x_dot - xr_dot;

V1 = e'*P*e + abs(Bstar(2,1))*(thx - Tx_star)'*inv(Gam_x)*(thx - Tx_star) + ...
              abs(Bstar(2,1))/Gam_r*(thr - Tr_star)^2;
dV2 = edot'*P*e + e'*P*edot + 2*abs(Bstar(2,1))*(thx - Tx_star)'*inv(Gam_x)*dthx + ...
                              2*abs(Bstar(2,1))/Gam_r*(thr - Tr_star)*dthr;

== matlab function AdaptiveControlsProjectPart1_Sethi/Reduced First Order System/MRC/controller ==
  data: r input; om input; vol output; tx_star parameter; tr_star parameter
%%%%%%%%%%%%%%%%%%%%%%%%%%%%%%%%%%%%%%%%%%%%%%%%%%%%%%%%%%%%%%%%%%%%%%%%%
%--- MRC, using star Controller (Without making the system adaptive) ---%
%%%%%%%%%%%%%%%%%%%%%%%%%%%%%%%%%%%%%%%%%%%%%%%%%%%%%%%%%%%%%%%%%%%%%%%%%
function vol = controller(r,om,tx_star, tr_star)
vol = tx_star*om + tr_star*r;     % vol is voltage

%%%%%%%%%%%%%%%%%%%%%%%%%%%%%%%%%%%%%%%%%%%%%%%%%%%%%%%%%%%%%%%%%%%%%%%%%
%--- MRC, using star Controller (Without making the system adaptive) ---%
%%%%%%%%%%%%%%%%%%%%%%%%%%%%%%%%%%%%%%%%%%%%%%%%%%%%%%%%%%%%%%%%%%%%%%%%%
% function vol = controller(r,om,tx, tr)
% vol = tx*om + tr*r;

== matlab function AdaptiveControlsProjectPart1_Sethi/Reduced First Order System/MRC/desired ==
  data: xd output; t input; r output; ar parameter; br parameter
function [xd,r] = desired(t,ar, br)

xd = 10*sin(2*t);
dxd = 20*cos(2*t);

r = (dxd - ar*xd)/br;

== matlab function AdaptiveControlsProjectPart1_Sethi/Reduced First Order System/MRC/plant ==
  data: om input; om_dot output; vol input; astar parameter; bstar parameter
function om_dot = plant(om,vol,astar, bstar)

om_dot = astar*om + bstar*vol;

== matlab function AdaptiveControlsProjectPart1_Sethi/Reduced First Order System/MRC/reference ==
  data: omr input; omr_dot output; r input; ar parameter; br parameter
function omr_dot = reference(omr,r,ar, br)

omr_dot = ar*omr + br*r;

== matlab function AdaptiveControlsProjectPart1_Sethi/Reduced First Order System/MRC/plant_Full2ndOrdersystem ==
  data: om input; om_dot output; vol input; J parameter; cur_dot output; B parameter; K parameter; L parameter; R parameter; cur input
function [om_dot, cur_dot] = plant(om,vol, J, B, K, L, R, cur)
% This is Assuming we did not know that Plant could be reduced to 1st order
% So we apply the full2nd order dynamic system in place of an approximated
% system
% Second order system !! Not assuming L = 0
om_dot = 1/J*(-B*om + K*cur);
cur_dot = 1/L*(-K*om - R*cur + vol);

% Note: The gains that worked for me were:
% ar = -10;   
% br = 10;
% 
% gam_x = 0.1;
% gam_r = 0.1;
% But obviously the theta_x and theta_r do not converge because I built a
% controller for a 1st order system but closing the loop with 2nd order
% system
% And you would notice that in the actual and reference trajectory graph
% that it never converges at some points, which most probably are the
% points where we have neglected L since it is too small but maybe the
% di/dt value is too large that it punishes us for our assumption of
% neglecting L

== matlab function AdaptiveControlsProjectPart1_Sethi/Full Second Order System/MRAC/With Projection/controllerSecondOrder ==
  data: r input; x input; vol output; thx input; thr input
%%%%%%%%%%%%%%%%%%%%%%%%%%%%%%%%%%%%%%%%%%
%--- MRAC, Making the system adaptive ---%
%%%%%%%%%%%%%%%%%%%%%%%%%%%%%%%%%%%%%%%%%%
% Vol = Tx*Om + Tr*r;
function vol = controller(r, x, thx, thr)
% vol = [Tx1 Tx2]*X + Tr*r;     % vol is voltage
vol = thx'*x + thr*r;                   % vol is voltage
% % Note: Tx and Tr are adaptive inputs taken in the simulink model so
% change them to "inputs" under "Model Explorer" in Simulink

% % Note: The gains that worked for me were:
% ar1 = -50; % Just tune these values
% ar2 = -40; % Just tune these values
% br = 10;
% Ar = [0, 1; ar1, ar2];   
% Br = [0; br];
% Gam_x = [.1 0; 0, .1];
% Gam_r = .1;

== matlab function AdaptiveControlsProjectPart1_Sethi/Full Second Order System/MRAC/With Projection/desiredSecondOrder ==
  data: dxd output; xd output; t input; r output; Ar parameter; Br parameter
function [dxd, xd,r] = desiredSecondOrder(t,Ar, Br)
xd = 10*sin(2*t);
dxd = 20*cos(2*t);
ddxd = -40*sin(2*t);

% r = (ddxd - ar1*xd - ar2*dxd)/br;
r = (ddxd - Ar(2,1)*xd - Ar(2,2)*dxd)/Br(2,1);

== matlab function AdaptiveControlsProjectPart1_Sethi/Full Second Order System/MRAC/With Projection/plantSecondOrder ==
  data: x input; xdot output; vol input; Astar parameter; Bstar parameter
%%%%%%%%%%%%%%%%%%%%%%%%%%%%%%%%%%%%%%%%%%
%--- MRAC, Making the system adaptive ---%
%%%%%%%%%%%%%%%%%%%%%%%%%%%%%%%%%%%%%%%%%%
% Vol = Tx*Om + Tr*r;
function xdot  = plantSecondOrder(x,vol, Astar, Bstar)
xdot = Astar*x + Bstar*vol;  % xdot = [0, 1; astar1 astar2]*x + [0; bstar]*vol;

== matlab function AdaptiveControlsProjectPart1_Sethi/Full Second Order System/MRAC/With Projection/referenceSecondOrder ==
  data: xr input; xr_dot output; r input; Ar parameter; Br parameter
function xr_dot = referenceSecondOrder(xr, r, Ar, Br)

% xr_dot = [0, 1; ar1, ar2]*xr + [0; br]*r;
xr_dot = Ar*xr + Br*r;

== matlab function AdaptiveControlsProjectPart1_Sethi/Full Second Order System/MRAC/Without Projection/adaptiveSecondOrder ==
  data: x input; xr input; r input; Gam_r parameter; Bstar parameter; Gam_x parameter; dthx output; dthr output; P2 parameter
%%%%%%%%%%%%%%%%%%%%%%%%%%%%%%%
%------WITHOUT PROJECTION-----%
%%%%%%%%%%%%%%%%%%%%%%%%%%%%%%%
function [dthx,dthr] = adaptive(x,xr,r,Gam_r, Bstar, Gam_x, P2)
% Adaptive Control Update Law
% Error dynamics
e = x - xr;

% Theta_x_dot and Theta_r_dot
% Note: Need to put e'*P2 in parenthesis because the result is a scalar and
% I want Matlab to multiple that scalar to Gam_x matrix and not Gam_x
% matrix to the vector e' first !!!
dthx = -Gam_x*(e'*P2)*x*sign(Bstar(2,1)); % dThx = -Gam_x*e'*P2*x*sign(bstar);
dthr = -Gam_r*(e'*P2)*r*sign(Bstar(2,1)); % dThr = -Gam_r*e'*P2*r*sign(bstar);

== matlab function AdaptiveControlsProjectPart1_Sethi/Full Second Order System/MRAC/Without Projection/controllerSecondOrder ==
  data: r input; x input; vol output; thx input; thr input
%%%%%%%%%%%%%%%%%%%%%%%%%%%%%%%%%%%%%%%%%%
%--- MRAC, Making the system adaptive ---%
%%%%%%%%%%%%%%%%%%%%%%%%%%%%%%%%%%%%%%%%%%
% Vol = Tx*Om + Tr*r;
function vol = controller(r, x, thx, thr)
% vol = [Tx1 Tx2]*X + Tr*r;     % vol is voltage
vol = thx'*x + thr*r;                   % vol is voltage
% % Note: Tx and Tr are adaptive inputs taken in the simulink model so
% change them to "inputs" under "Model Explorer" in Simulink

% % Note: The gains that worked for me were:
% ar1 = -100; % Just tune these values
% ar2 = -80; % Just tune these values
% br = 80;
% Ar = [0, 1; ar1, ar2];   
% Br = [0; br];
% Gam_x = [.1 0; 0, .1];
% Gam_r = .1;

== matlab function AdaptiveControlsProjectPart1_Sethi/Full Second Order System/MRAC/Without Projection/desiredSecondOrder ==
  data: dxd output; xd output; t input; r output; Ar parameter; Br parameter
% function [ddxd, dxd, xd,r] = desiredSecondOrder(t,Ar, Br)
function [dxd, xd,r] = desiredSecondOrder(t,Ar, Br)
xd = 10*sin(2*t);
dxd = 20*cos(2*t);
ddxd = -40*sin(2*t);

% r = (ddxd - ar1*xd - ar2*dxd)/br;
r = (ddxd - Ar(2,1)*xd - Ar(2,2)*dxd)/Br(2,1);

== matlab function AdaptiveControlsProjectPart1_Sethi/Full Second Order System/MRAC/Without Projection/lyapunov ==
  data: x input; xr input; r input; V1 output; thx input; thr input; dV2 output; dV3 output; P parameter; Q parameter; Gam_x parameter; Gam_r parameter; Astar parameter; Br parameter; Tx_star parameter; Tr_star parameter; Bstar parameter; Ar parameter
function [V1,dV2,dV3] = lyapunov(x,xr,r,thx,thr,P,Q,Gam_x,Gam_r,...
                                 Astar,Br,Tx_star, Tr_star, Bstar, Ar)

P2 = P(:,2);

e = x - xr;
dV3= -e'*Q*e;

dthx = -Gam_x*(e'*P2)*x*sign(Bstar(2,1)); % -Gam_x*(e'*P2)*x*sign(bstar);
dthr = -Gam_r*(e'*P2)*r*sign(Bstar(2,1)); % -gam_r*(e'*P2)*r*sign(bstar);

vol = thx'*x + thr*r;
 
xr_dot = Ar*xr + Br*r;    % Ar*xr + [0 ; br]*r; 
x_dot = Astar*x + Bstar*vol; % [0 1;astar1 astar2]*x + [0 ; bstar]*vol;
edot= x_dot - xr_dot;

V1 = e'*P*e + abs(Bstar(2,1))*(thx - Tx_star)'*inv(Gam_x)*(thx - Tx_star) + ...
              abs(Bstar(2,1))/Gam_r*(thr - Tr_star)^2;
dV2 = edot'*P*e + e'*P*edot + 2*abs(Bstar(2,1))*(thx - Tx_star)'*inv(Gam_x)*dthx + ...
                              2*abs(Bstar(2,1))/Gam_r*(thr - Tr_star)*dthr;

== matlab function AdaptiveControlsProjectPart1_Sethi/Full Second Order System/MRAC/Without Projection/plantSecondOrder ==
  data: x input; xdot output; vol input; Astar parameter; Bstar parameter
%%%%%%%%%%%%%%%%%%%%%%%%%%%%%%%%%%%%%%%%%%%%%%%%%%%%%%%%%%%%%%%%%%%%%%%%%
%--- MRC, using star Controller (Without making the system adaptive) ---%
%%%%%%%%%%%%%%%%%%%%%%%%%%%%%%%%%%%%%%%%%%%%%%%%%%%%%%%%%%%%%%%%%%%%%%%%%

function xdot  = plantSecondOrder(x,vol, Astar, Bstar)
% Note: vol is your control effort u
xdot = Astar*x + Bstar*vol;  % xdot = [0, 1; astar1 astar2]*x + [0; bstar]*vol;
%om_dot = [1 0]*xdot;


%%%%%%%%%%%%%%%%%%%%%%%%%%%%%%%%%%%%%%%%%%
%--- MRAC, Making the system adaptive ---%
%%%%%%%%%%%%%%%%%%%%%%%%%%%%%%%%%%%%%%%%%%
% Vol = Tx*Om + Tr*r;
% function xdot  = plantSecondOrder(x,vol, Astar, Bstar)
% xdot = Astar*x + Bstar*vol;  % xdot = [0, 1; astar1 astar2]*x + [0; bstar]*vol;

== matlab function AdaptiveControlsProjectPart1_Sethi/Full Second Order System/MRAC/Without Projection/referenceSecondOrder ==
  data: xr input; xr_dot output; r input; Ar parameter; Br parameter
function xr_dot = referenceSecondOrder(xr, r, Ar, Br)

% xr_dot = [0, 1; ar1, ar2]*xr + [0; br]*r;
xr_dot = Ar*xr + Br*r;
